simulink model "PID_Tuning_Ideal_Feedback_Control"  (R2025b)
settings: Solver=FixedStepAuto  StartTime=0.0  StopTime=tspan  FixedStep=dt_sim  RelTol=rel_tol  AbsTol=abs_tol
undefined symbols (not defined in the file): battery_voltage
settings Model: Creator=koryh  LastModifiedBy=koryh

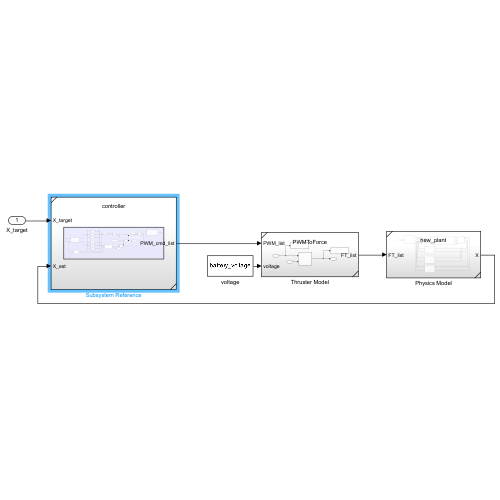
[thumbnail: Simulink's stored preview of the top-level diagram]
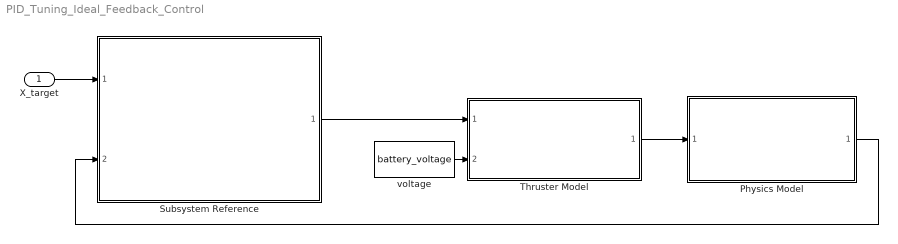
== system PID_Tuning_Ideal_Feedback_Control ==
  X_target : Inport
  Physics Model : Subsystem  ReferencedSubsystem=new_plant
  Subsystem Reference : Subsystem  ReferencedSubsystem=controller
  Thruster Model : Subsystem  ReferencedSubsystem=PWMToForce
  voltage : Constant  Value=battery_voltage
  wires:
  Thruster Model/1 -> Physics Model/1
  voltage/1 -> Thruster Model/2
  Physics Model/1 -> Subsystem Reference/2
  Subsystem Reference/1 -> Thruster Model/1
  X_target/1 -> Subsystem Reference/1
